simulink model "frequence_response_2"  (R2021b)
settings: Solver=VariableStepAuto  StartTime=0.0  StopTime=30  RelTol=1e-3
values from neighbouring files (symbols this model uses):
  f2 = [0 2]    [main.m]    (also in main1.m)
  phi2 = [0 0]    [main.m]    (also in main1.m)
  U2_max = [4 6]    [main.m]    (also in main1.m)
undefined symbols (not defined in the file or in its folder): A, B, C, D
settings Model: Creator=PaoloA  LastModifiedBy=PaoloA

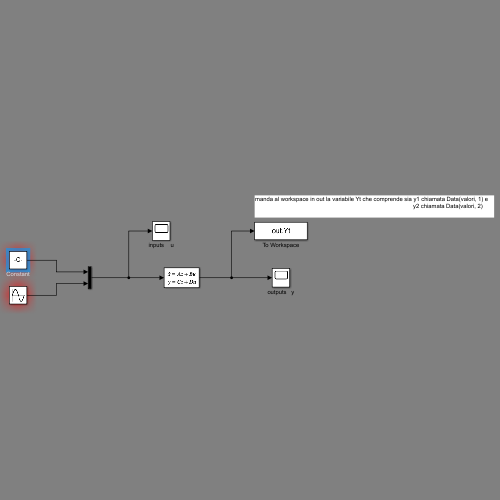
[thumbnail: Simulink's stored preview of the top-level diagram]
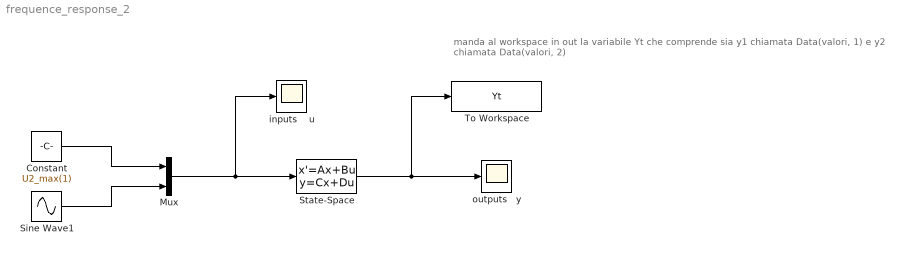
== system frequence_response_2 ==
  note: manda al workspace in out la variabile Yt che comprende sia y1 chiamata Data(valori, 1) e
      | 												           y2 chiamata Data(valori, 2)
  Constant : Constant  Value=U2_max(1)
  Mux : Mux  Inputs=2
  Sine Wave1 : Sin  Amplitude=U2_max(2)  Frequency=f2(2)  Phase=phi2(2)  SampleTime=0
  State-Space : StateSpace  A=A  B=B  C=C  D=D  InitialCondition=0
  To Workspace : ToWorkspace  VariableName=Yt  SaveFormat=Timeseries  SampleTime=-1
  inputs    u : Scope
  outputs   y : Scope
  wires:
  State-Space/1 -> To Workspace/1, outputs   y/1
  Mux/1 -> inputs    u/1, State-Space/1
  Constant/1 -> Mux/1
  Sine Wave1/1 -> Mux/2
